simulink model "scm"  (R2020a)
settings: Solver=VariableStepAuto  StartTime=0.0  StopTime=150.0  RelTol=1e-3
values from neighbouring files (symbols this model uses):
  alpha = 0.1    [scm.m]
  alpha1 = 0.01    [scm.m]
  d = L-1    (= 2)    [scm.m]
  k = norminv(CLS)    [scm.m]
  L = 3    [scm.m]
  S = 1000    [scm.m]
  SIGMAk = sqrt(L)*sqrt(1+(alpha*(L-1))+((1/6)*(alpha^.2)*(L-1)*((2*L)-1)))    [scm.m]
undefined symbols (not defined in the file or in its folder): magnitude
settings Model: Creator=Houda Assad  LastModifiedBy=Houda Assad

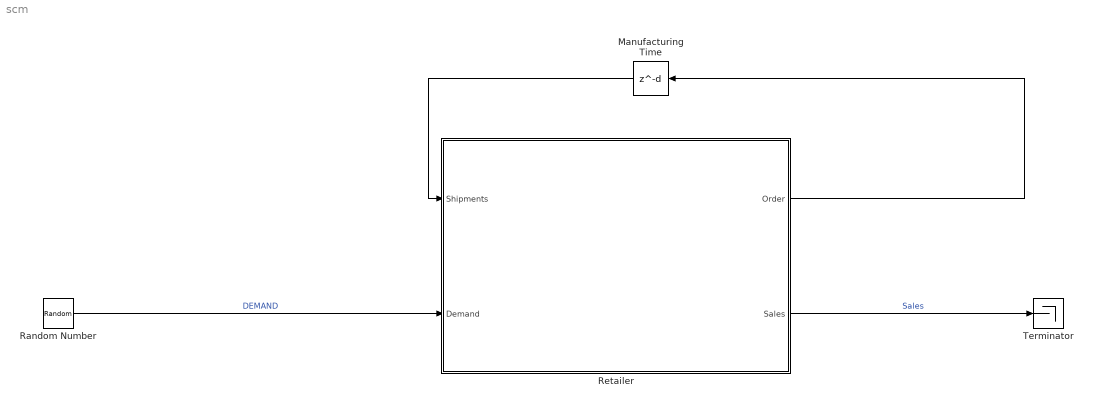
== system scm ==
  Manufacturing Time : Delay  DelayLength=d
  "Random Number  " : RandomNumber  Mean=100  Variance=20  Seed=.1  SampleTime=0.5
  Retailer : Subsystem
  Terminator : Terminator
  wires:
  Manufacturing Time/1 -> Retailer/1(Shipments)
  Retailer/1(Order) -> Manufacturing Time/1
  Retailer/2(Sales) -> Terminator/1  "Sales"
  "Random Number  "/1 -> Retailer/2(Demand)  "DEMAND"

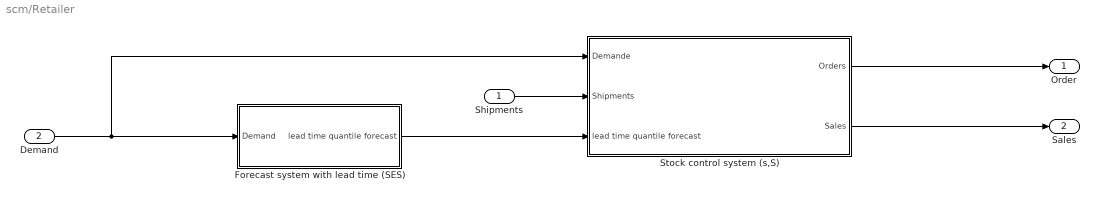
== system scm/Retailer ==
  Shipments : Inport
  Demand : Inport  Port=2
  Forecast system with lead time (SES) : Subsystem
  Stock control system (s,S) : Subsystem
  Order : Outport
  Sales : Outport  Port=2
  wires:
  Demand/1 -> Forecast system with lead time (SES)/1(Demand), Stock control system (s,S)/1("Demande ")
  Stock control system (s,S)/1("Orders ") -> Order/1
  Shipments/1 -> Stock control system (s,S)/2(Shipments)
  Stock control system (s,S)/2(Sales) -> Sales/1
  Forecast system with lead time (SES)/1("lead time quantile forecast ") -> Stock control system (s,S)/3("lead time quantile forecast ")

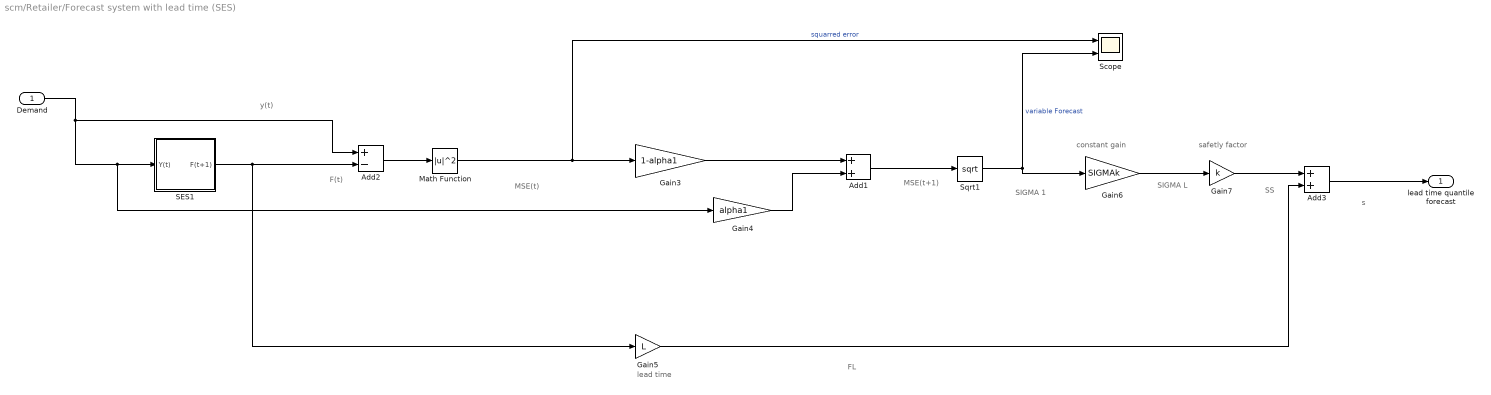
== system scm/Retailer/Forecast system with lead time (SES) ==
  note: SIGMA 1
  note: safetly factor
  note: s
  note: SIGMA L
  note: SS
  note: MSE(t)
  note: F(t)
  note: y(t)
  note: lead time
  note: FL
  note: MSE(t+1)
  note: constant gain
  Demand : Inport
  Add1 : Sum
  Add2 : Sum  Inputs=+-
  Add3 : Sum
  Gain3 : Gain  Gain=1-alpha1
  Gain4 : Gain  Gain=alpha1
  Gain5 : Gain  Gain=L
  Gain6 : Gain  Gain=SIGMAk
  Gain7 : Gain  Gain=k
  Math Function : Math  Operator=magnitude^2  SaturateOnIntegerOverflow=on
  SES1 : Subsystem
  "Scope " : Scope  NumInputPorts=2
  Sqrt1 : Sqrt  SaturateOnIntegerOverflow=on
  "lead time quantile forecast " : Outport
  wires:
  Gain6/1 -> Gain7/1
  SES1/1(F(t+1)) -> Gain5/1, Add2/2
  Sqrt1/1 -> "Scope "/2, Gain6/1  "variable Forecast"
  Add3/1 -> "lead time quantile forecast "/1
  Add1/1 -> Sqrt1/1
  Gain4/1 -> Add1/2
  Gain7/1 -> Add3/1
  Math Function/1 -> "Scope "/1, Gain3/1  "squarred error"
  Demand/1 -> Add2/1, Gain4/1, SES1/1(Y(t))
  Gain5/1 -> Add3/2
  Gain3/1 -> Add1/1
  Add2/1 -> Math Function/1

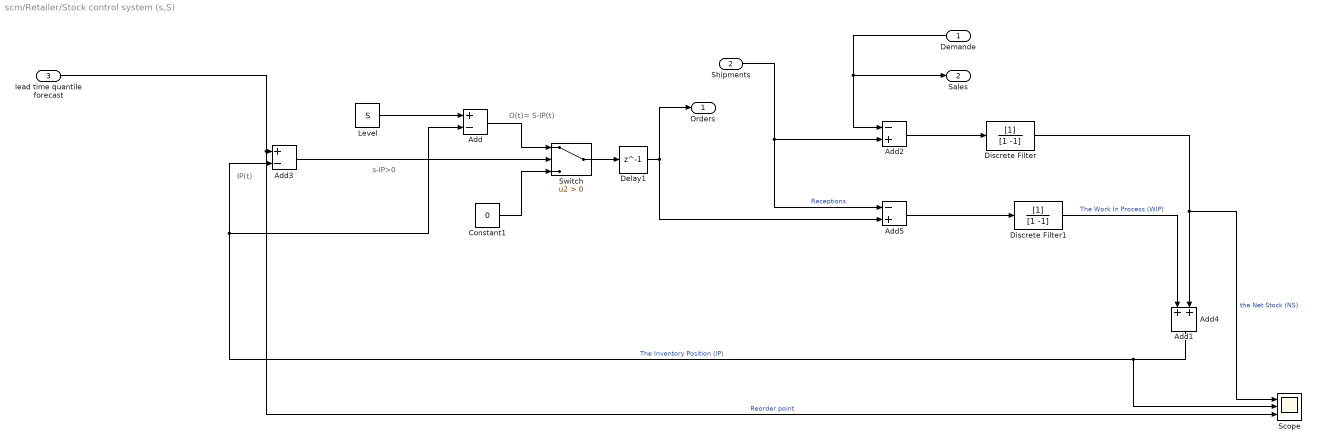
== system scm/Retailer/Stock control system (s,S) ==
  note: s-IP>0
  note: O(t)= S-IP(t)
  note: IP(t)
  "Demande " : Inport
  Shipments : Inport  Port=2
  "lead time quantile forecast " : Inport  Port=3
  Add : Sum  Inputs=+-
  Add1 : Sum
  Add2 : Sum  Inputs=-+
  Add3 : Sum  Inputs=+-
  Add4 : Sum
  Add5 : Sum  Inputs=-+
  Constant1 : Constant  Value=0
  Delay1 : Delay  DelayLength=1
  Discrete Filter : DiscreteFilter  Denominator=[1 -1]  InitialStates=400
  Discrete Filter1 : DiscreteFilter  Denominator=[1 -1]
  Level : Constant  Value=S
  Scope : Scope  NumInputPorts=3
  "Switch " : Switch  Criteria=u2 > Threshold
  "Orders " : Outport
  Sales : Outport  Port=2
  wires:
  Discrete Filter1/1 -> Add4/1  "The Work In Process (WIP)"
  Add3/1 -> "Switch "/2
  Level/1 -> Add/1
  Add5/1 -> Discrete Filter1/1
  "lead time quantile forecast "/1 -> Scope/3, Add3/1  "Reorder point"
  Delay1/1 -> "Orders "/1, Add5/2
  Add/1 -> "Switch "/1
  "Demande "/1 -> Sales/1, Add2/1
  Shipments/1 -> Add5/1, Add2/2  "Receptions"
  Constant1/1 -> "Switch "/3
  Add2/1 -> Discrete Filter/1
  Discrete Filter/1 -> Add4/2, Scope/1  "the Net Stock (NS)"
  "Switch "/1 -> Delay1/1
  Add4/1 -> Scope/2, Add/2, Add3/2  "The Inventory Position (IP)"

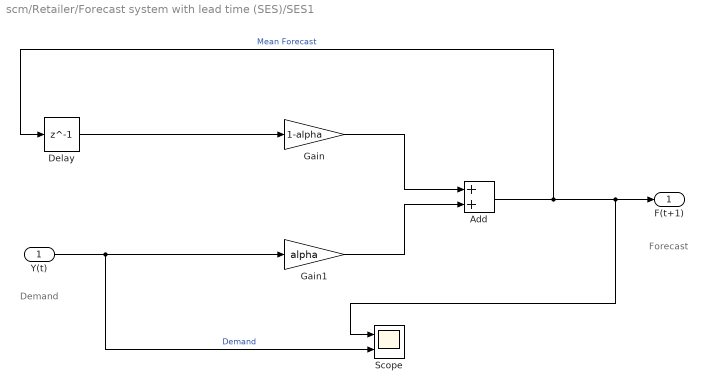
== system scm/Retailer/Forecast system with lead time (SES)/SES1 ==
  note: Demand
  note: Forecast
  Y(t) : Inport
  "Add " : Sum
  "Delay " : Delay  DelayLength=1
  "Gain " : Gain  Gain=1-alpha
  "Gain1 " : Gain  Gain=alpha
  Scope : Scope  NumInputPorts=2
  F(t+1) : Outport
  wires:
  Y(t)/1 -> Scope/2, "Gain1 "/1  "Demand"
  "Add "/1 -> Scope/1, F(t+1)/1, "Delay "/1  "Mean Forecast"
  "Delay "/1 -> "Gain "/1
  "Gain "/1 -> "Add "/1
  "Gain1 "/1 -> "Add "/2
